simulink model "sSpiegelIad"  (R2012b)
settings: Solver=ode45  StartTime=0.0  StopTime=10.0  RelTol=1e-3
values from neighbouring files (symbols this model uses):
  J = J*1e-2*1e-2    (= 9.33e-12)    [msSpiegel.m]    (also in msSpiegel_PID.m = 9.33e-08; msSpiegel_Pad.m = 9.33e-08; msSpiegel_Pad_Neue_Werte.m = 9.33e-09; msSpiegel_Pad_Neue_Werte_Strom.m = 9.33e-10)
  KMPHI = 35e-3    (= 0.035)    [msSpiegel.m]    (also in msSpiegel_PID.m = 0.063; msSpiegel_Pad.m = 0.063; msSpiegel_Pad_Neue_Werte.m; msSpiegel_Pad_Neue_Werte_Strom.m)
  LA = 10e-6    (= 1e-05)    [msSpiegel.m]    (also in msSpiegel_PID.m = 0.000448; msSpiegel_Pad.m = 0.000448; msSpiegel_Pad_Neue_Werte.m = 3e-06; msSpiegel_Pad_Neue_Werte_Strom.m = 3e-06)
  Mspiegel = 130.25e-6    (= 0.00013025)    [msSpiegel.m]    (also in msSpiegel_PID.m = 0.13025; msSpiegel_Pad.m = 0.13025; msSpiegel_Pad_Neue_Werte_Strom.m = 3.025e-05)
  phi = 0.4    [Sensor_initieren.m]    (also in msSpiegel.m = 0.349065850399; msSpiegel_PID.m = 0.349065850399; msSpiegel_Pad.m = 0.349065850399; msSpiegel_Pad_Neue_Werte.m = 0.349065850399)
  r = []    [faltungsfunktionen.m]    (also in faltungsfunktionen3.m; msSpiegel.m = 6e-06; msSpiegel_PID.m = 6e-05; msSpiegel_Pad.m = 6e-05)
  RA = 0.1    [msSpiegel.m]    (also in msSpiegel_PID.m = 0.16; msSpiegel_Pad.m = 0.16; msSpiegel_Pad_Neue_Werte.m; msSpiegel_Pad_Neue_Werte_Strom.m)
settings Model: Creator=froriep  LastModifiedBy=michamann
settings DataIOCC: SignalLoggingSaveFormat=ModelDataLogs
settings DebuggingCC: FcnCallInpInsideContextMsg=EnableAllAsWarning
settings GRTTargetCC: CombineOutputUpdateFcns=off  GRTInterface=on

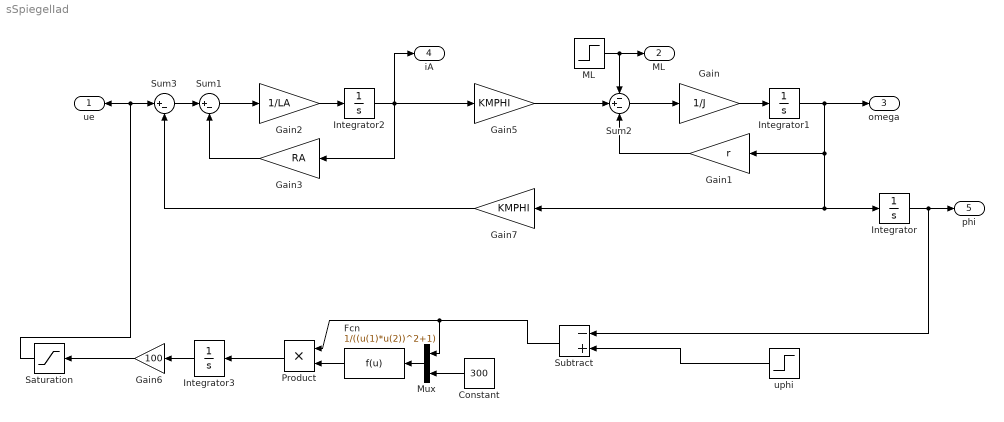
== system sSpiegelIad ==
  Constant : Constant  Value=300
  Fcn : Fcn  Expr=1/((u(1)*u(2))^2+1)
  Gain : Gain  Gain=1/J
  Gain1 : Gain  Gain=r
  Gain2 : Gain  Gain=1/LA
  Gain3 : Gain  Gain=RA
  Gain5 : Gain  Gain=KMPHI
  Gain6 : Gain  Gain=100
  Gain7 : Gain  Gain=KMPHI
  Integrator : Integrator
  Integrator1 : Integrator
  Integrator2 : Integrator
  Integrator3 : Integrator  UpperSaturationLimit=24  LowerSaturationLimit=-24
  ML : Step  Time=0  After=Mspiegel  SampleTime=0
  Mux : Mux  Inputs=2
  Product : Product  RndMeth=Zero  InputSameDT=on
  Saturation : Saturate
  Subtract : Sum  Inputs=-+
  Sum1 : Sum  Inputs=|+-
  Sum2 : Sum  Inputs=-+-
  Sum3 : Sum  Inputs=|+-
  uphi : Step  Time=100  Before=phi  After=phi  SampleTime=0
  "ue " : Outport
  "ML " : Outport  Port=2
  omega : Outport  Port=3
  iA : Outport  Port=4
  phi : Outport  Port=5
  wires:
  Integrator1/1 -> Integrator/1, Gain7/1, Gain1/1, omega/1
  Gain/1 -> Integrator1/1
  Sum2/1 -> Gain/1
  Gain1/1 -> Sum2/3
  Integrator2/1 -> Gain3/1, Gain5/1, iA/1
  Gain2/1 -> Integrator2/1
  Sum1/1 -> Gain2/1
  Gain5/1 -> Sum2/2
  ML/1 -> Sum2/1, "ML "/1
  Sum3/1 -> Sum1/1
  Gain3/1 -> Sum1/2
  Gain7/1 -> Sum3/2
  Integrator/1 -> Subtract/1, phi/1
  uphi/1 -> Subtract/2
  Subtract/1 -> Mux/1, Product/1
  Fcn/1 -> Product/2
  Constant/1 -> Mux/2
  Mux/1 -> Fcn/1
  Integrator3/1 -> Gain6/1
  Product/1 -> Integrator3/1
  Gain6/1 -> Saturation/1
  Saturation/1 -> Sum3/1, "ue "/1
